simulink model "QCM"  (R2020b)
settings: Solver=VariableStepAuto  StartTime=0.0  StopTime=10.0  RelTol=1e-3
undefined symbols (not defined in the file or in its folder): par
libraries: simulink x1
settings Model: Creator=maart  LastModifiedBy=maart
settings SolverCC: ZeroCrossAlgorithm=Adaptive
settings DebuggingCC: IgnoredZcDiagnostic=none

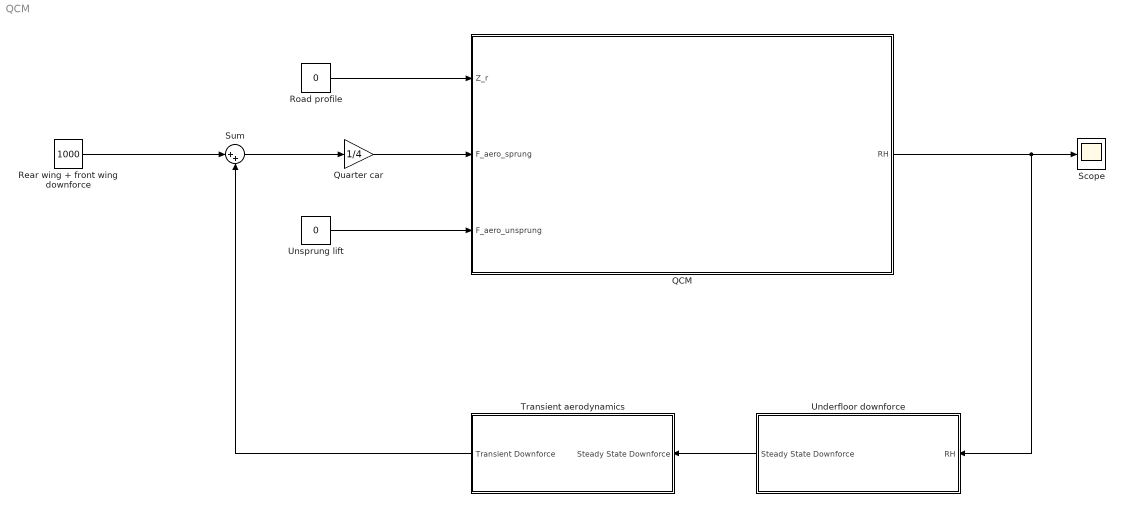
== system QCM ==
  QCM : Subsystem
  Quarter car : Gain  Gain=1/4
  Rear wing + front wing downforce : Constant  Value=1000
  Road profile : Constant  Value=0
  Scope : Scope
  Sum : Sum  Inputs=|++
  Transient aerodynamics : Subsystem
  Underfloor downforce : Subsystem
  Unsprung lift : Constant  Value=0
  wires:
  Road profile/1 -> QCM/1(Z_r)
  Unsprung lift/1 -> QCM/3(F_aero_unsprung)
  QCM/1(RH) -> Scope/1, Underfloor downforce/1(RH)
  Underfloor downforce/1(Steady State Downforce) -> Transient aerodynamics/1(Steady State Downforce)
  Rear wing + front wing downforce/1 -> Sum/1
  Transient aerodynamics/1(Transient Downforce) -> Sum/2
  Sum/1 -> Quarter car/1
  Quarter car/1 -> QCM/2(F_aero_sprung)

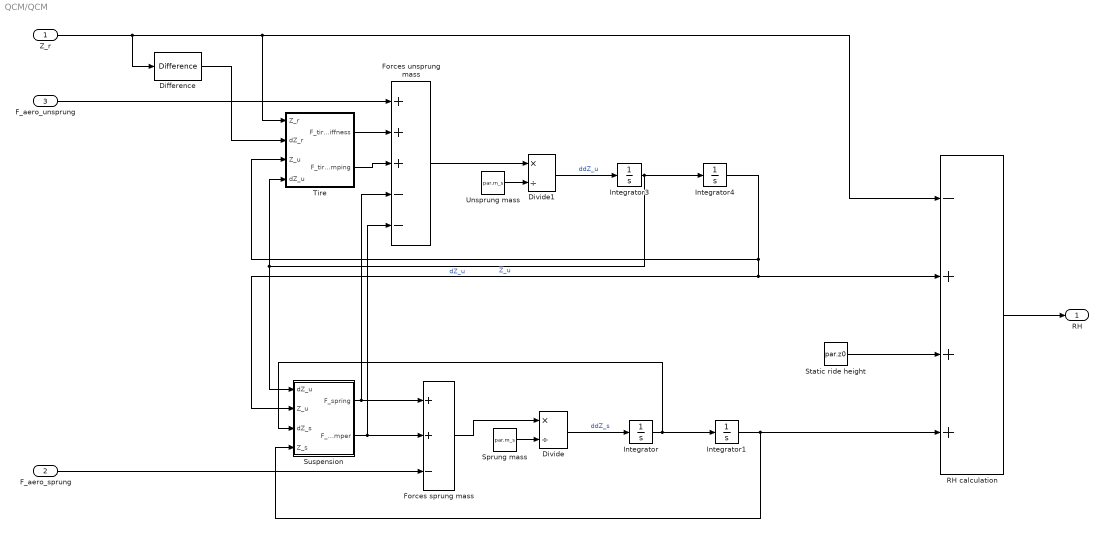
== system QCM/QCM ==
  Z_r : Inport
  F_aero_sprung : Inport  Port=2
  F_aero_unsprung : Inport  Port=3
  Difference : simulink/Discrete/Difference  ICPrevInput=0.0  OutMin=[]  OutMax=[]  OutDataType=fixdt(1, 16)  OutScaling=2^-10  DoSatur=off
  Divide : Product  Inputs=*/
  Divide1 : Product  Inputs=*/
  Forces sprung mass : Sum  Inputs=++-
  Forces unsprung mass : Sum  Inputs=+++--
  Integrator{,1,3..4} (4 alike) : Integrator
  RH calculation : Sum  Inputs=-+++
  Sprung mass : Constant  Value=par.m_s
  Static ride height : Constant  Value=par.z0
  Suspension : Subsystem
  Tire : Subsystem
  Unsprung mass : Constant  Value=par.m_s
  RH : Outport
  wires:
  Forces sprung mass/1 -> Divide/1
  Sprung mass/1 -> Divide/2
  Divide/1 -> Integrator/1  "ddZ_s"
  Integrator/1 -> Suspension/3(dZ_s), Integrator1/1
  Integrator1/1 -> Suspension/4(Z_s), RH calculation/4
  F_aero_sprung/1 -> Forces sprung mass/3
  Integrator3/1 -> Integrator4/1, Tire/4(dZ_u), Suspension/1(dZ_u)  "dZ_u"
  Integrator4/1 -> Tire/3(Z_u), Suspension/2(Z_u), RH calculation/2  "Z_u"
  Unsprung mass/1 -> Divide1/2
  Divide1/1 -> Integrator3/1  "ddZ_u"
  Forces unsprung mass/1 -> Divide1/1
  Static ride height/1 -> RH calculation/3
  Z_r/1 -> Difference/1, Tire/1(Z_r), RH calculation/1
  RH calculation/1 -> RH/1
  Suspension/1(F_spring) -> Forces unsprung mass/4, Forces sprung mass/1
  Suspension/2(F_damper) -> Forces sprung mass/2, Forces unsprung mass/5
  Tire/2(F_tire_damping) -> Forces unsprung mass/3
  Tire/1(F_tire_stiffness) -> Forces unsprung mass/2
  F_aero_unsprung/1 -> Forces unsprung mass/1
  Difference/1 -> Tire/2(dZ_r)

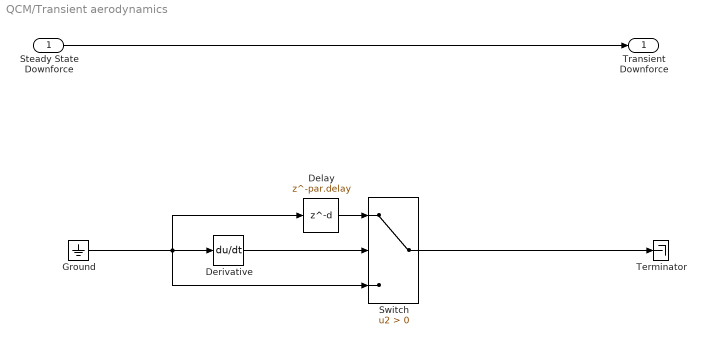
== system QCM/Transient aerodynamics ==
  Steady State Downforce : Inport
  Delay : Delay  DelayLength=par.delay  InitialCondition=par.initial_downforce
  Derivative : Derivative
  Ground : Ground
  Switch : Switch  Criteria=u2 > Threshold
  Terminator : Terminator
  Transient Downforce : Outport
  wires:
  Switch/1 -> Terminator/1
  Delay/1 -> Switch/1
  Derivative/1 -> Switch/2
  Ground/1 -> Switch/3, Delay/1, Derivative/1
  Steady State Downforce/1 -> Transient Downforce/1

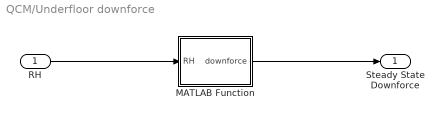
== system QCM/Underfloor downforce ==
  RH : Inport
  MATLAB Function : MATLAB Function  TreatAsAtomicUnit=on
  Steady State Downforce : Outport
  wires:
  RH/1 -> MATLAB Function/1(RH)
  MATLAB Function/1(downforce) -> Steady State Downforce/1

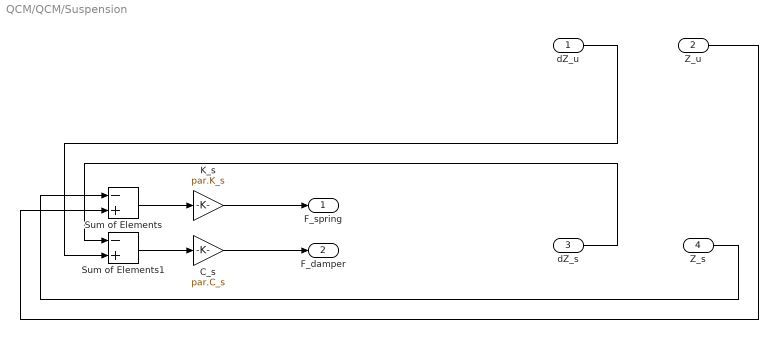
== system QCM/QCM/Suspension ==
  dZ_u : Inport
  Z_u : Inport  Port=2
  dZ_s : Inport  Port=3
  Z_s : Inport  Port=4
  C_s : Gain  Gain=par.C_s
  K_s : Gain  Gain=par.K_s
  Sum of Elements : Sum  Inputs=-+
  Sum of Elements1 : Sum  Inputs=-+
  F_spring : Outport
  F_damper : Outport  Port=2
  wires:
  Z_s/1 -> Sum of Elements/1
  Sum of Elements/1 -> K_s/1
  Sum of Elements1/1 -> C_s/1
  K_s/1 -> F_spring/1
  dZ_u/1 -> Sum of Elements1/2
  Z_u/1 -> Sum of Elements/2
  C_s/1 -> F_damper/1
  dZ_s/1 -> Sum of Elements1/1

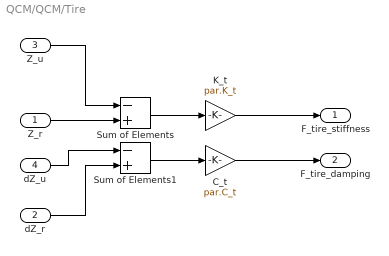
== system QCM/QCM/Tire ==
  Z_r : Inport
  dZ_r : Inport  Port=2
  Z_u : Inport  Port=3
  dZ_u : Inport  Port=4
  C_t : Gain  Gain=par.C_t
  K_t : Gain  Gain=par.K_t
  Sum of Elements : Sum  Inputs=-+
  Sum of Elements1 : Sum  Inputs=-+
  F_tire_stiffness : Outport
  F_tire_damping : Outport  Port=2
  wires:
  Sum of Elements/1 -> K_t/1
  Sum of Elements1/1 -> C_t/1
  K_t/1 -> F_tire_stiffness/1
  C_t/1 -> F_tire_damping/1
  Z_u/1 -> Sum of Elements/1
  Z_r/1 -> Sum of Elements/2
  dZ_u/1 -> Sum of Elements1/1
  dZ_r/1 -> Sum of Elements1/2

== matlab function QCM/Underfloor downforce/MATLAB Function ==
  data: RH input; downforce output
function downforce = fcn(RH)
    RH_crit = 10;
    if RH<RH_crit
        downforce = 10*RH;
    else
        downforce = 10000/(RH+0.001);
    end
end
